simulink model "ES101A_DiagcMgr"  (R2013b)
settings: Solver=ode45  StartTime=0.0  StopTime=0.44  RelTol=1e-3
values from neighbouring files (symbols this model uses):
  BrdgVltg = DataDict.IpSignal    [ES101A_DiagcMgr_DataDict.m]
  DEM_CLEAR_PENDING = DataDict.Constant    [ES101A_DiagcMgr_DataDict.m]
  DEM_DTC_GROUP_ALL_DTCS = DataDict.Constant    [ES101A_DiagcMgr_DataDict.m]
  DFTAGICNTR_CNT_U08 = DataDict.Constant    [ES101A_DiagcMgr_DataDict.m]
  DIAGCMGR_NTCINFOSTSTESTFAILD_CNT_U08 = DataDict.Constant    [ES101A_DiagcMgr_DataDict.m]
  DIAGCMGR_NTCINFOSTSTESTFAILDTHISIGNCYC_CNT_U08 = DataDict.Constant    [ES101A_DiagcMgr_DataDict.m]
  DIAGCMGR_NTCINFOSTSTESTNOTCMPLTHISIGNCYC_CNT_U08 = DataDict.Constant    [ES101A_DiagcMgr_DataDict.m]
  DiagcMgrFltResp = DataDict.Calibration    [ES101A_DiagcMgr_DataDict.m]
  DiagcMgrNtcFltAry = DataDict.NVM    [ES101A_DiagcMgr_DataDict.m]
  DIAGCSTSCTRLDSHTDWNFLTPRSNT_CNT_U16 = DataDict.Constant    [ES101A_DiagcMgr_DataDict.m]
  DIAGCSTSDFTHWAG_CNT_U16 = DataDict.Constant    [ES101A_DiagcMgr_DataDict.m]
  DIAGCSTSDFTHWAGSERLCOMEXPRTVAL_CNT_U16 = DataDict.Constant    [ES101A_DiagcMgr_DataDict.m]
  DIAGCSTSDFTVEHSPD_CNT_U16 = DataDict.Constant    [ES101A_DiagcMgr_DataDict.m]
  DIAGCSTSININVAL_CNT_U16 = DataDict.Constant    [ES101A_DiagcMgr_DataDict.m]
  DIAGCSTSIVTR1INACTV_CNT_U16 = DataDict.Constant    [ES101A_DiagcMgr_DataDict.m]
  DIAGCSTSIVTR2INACTV_CNT_U16 = DataDict.Constant    [ES101A_DiagcMgr_DataDict.m]
  DIAGCSTSLIMDTPRFMNC_CNT_U16 = DataDict.Constant    [ES101A_DiagcMgr_DataDict.m]
  DIAGCSTSRAMPTOZEROFLTPRSNT_CNT_U16 = DataDict.Constant    [ES101A_DiagcMgr_DataDict.m]
  DIAGCSTSWHLIMBREJCTNDI_CNT_U16 = DataDict.Constant    [ES101A_DiagcMgr_DataDict.m]
  DTCIDXSTSFAIL_CNT_U08 = DataDict.Constant    [ES101A_DiagcMgr_DataDict.m]
  DTCIDXSTSNONTC_CNT_U08 = DataDict.Constant    [ES101A_DiagcMgr_DataDict.m]
  DTCIDXSTSNORES_CNT_U08 = DataDict.Constant    [ES101A_DiagcMgr_DataDict.m]
  DTCIDXSTSPASS_CNT_U08 = DataDict.Constant    [ES101A_DiagcMgr_DataDict.m]
  DTCIDXSTSUPDCFMD_CNT_U08 = DataDict.Constant    [ES101A_DiagcMgr_DataDict.m]
  ELECGLBPRM_IVTRCNT_CNT_U08 = DataDict.ConfigParam    [ES101A_DiagcMgr_DataDict.m]
  FLTINJ_DIAGCMGR_DIAGCSTSIVTR1INACTV = DataDict.Constant    [ES101A_DiagcMgr_DataDict.m]
  FLTINJ_DIAGCMGR_DIAGCSTSIVTR2INACTV = DataDict.Constant    [ES101A_DiagcMgr_DataDict.m]
  HwTq = DataDict.IpSignal    [ES101A_DiagcMgr_DataDict.m]
  IgnCntr = DataDict.IpSignal    [ES101A_DiagcMgr_DataDict.m]
  MAXDEBCNTRVAL_CNT_S16 = DataDict.Constant    [ES101A_DiagcMgr_DataDict.m]
  MAXRAMPRATE_ULSPERSEC_F32 = DataDict.Constant    [ES101A_DiagcMgr_DataDict.m]
  MINDEBCNTRVAL_CNT_S16 = DataDict.Constant    [ES101A_DiagcMgr_DataDict.m]
  MINRAMPRATE_ULSPERSEC_F32 = DataDict.Constant    [ES101A_DiagcMgr_DataDict.m]
  SCAMOTTQCMDTOONE_ULS_F32 = DataDict.Constant    [ES101A_DiagcMgr_DataDict.m]
  SCAMOTTQCMDTOZERO_ULS_F32 = DataDict.Constant    [ES101A_DiagcMgr_DataDict.m]
  SysSt = DataDict.IpSignal    [ES101A_DiagcMgr_DataDict.m]
  VehSpd = DataDict.IpSignal    [ES101A_DiagcMgr_DataDict.m]
undefined symbols (not defined in the file or in its folder): ActvMotTqCmdSca, ActvRampRate, AgiCntr, Dem_DTCFormatType, Dem_DTCOriginType, Dem_EventStatusType, DiagcData, DiagcMgrNtcMap, DiagcSts, DtcEnaMask, EcuT, HistNtcFltAry, MicroDiagcData, MotTq, NtcNr, NtcNrWithResd1, NtcStInfo, ProxySetNtcData, Sts, SysSt1, TOTNROFDTC_CNT_U08
libraries: simulink x151, FloatToFixd x5, NxtrNvM x4
(part 11 of 13)

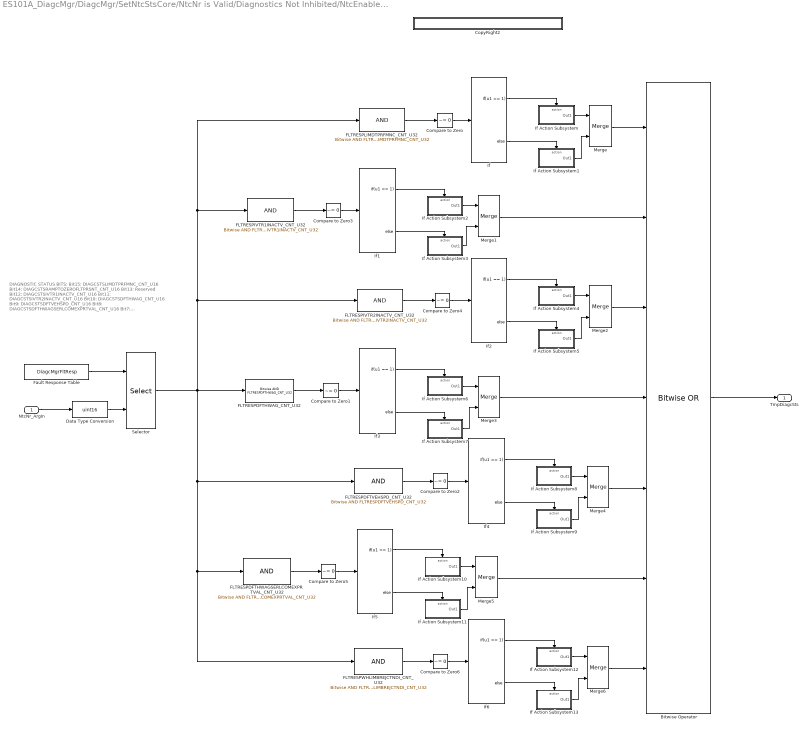
== system ES101A_DiagcMgr/DiagcMgr/SetNtcStsCore/NtcNr is Valid/Diagnostics Not Inhibited/NtcEnabled/NTCSTS_PREFAILD/Update NtcInfoSts, DebCntr and Process RampRate/DebCntr = MAXDEBCNTRVAL_CNT_S16/ProcessRampResponse and DiagcSts/ProcessDiagcSts ==
  note: DIAGNOSTIC  STATUS  BITS:
      |
      | Bit15: DIAGCSTSLIMDTPRFMNC_CNT_U16
      | Bit14: DIAGCSTSRAMPTOZEROFLTPRSNT_CNT_U16
      | Bit13: Reserved
      | Bit12: DIAGCSTSIVTR1INACTV_CNT_U16
      | Bit11: DIAGCSTSIVTR2INACTV_CNT_U16
      | Bit10: DIAGCSTSDFTHWAG_CNT_U16
      | Bit9:   DIAGCSTSDFTVEHSPD_CNT_U16
      | Bit8:   DIAGCSTSDFTHWAGSERLCOMEXPRTVAL_CNT_U16
      | Bit7:   DIAGCSTSWHLIMBREJCTNDI_CNT_U16
      | Bit6:	   DIAGCSTSCTRLDIRAMP_CNT_U16
  NtcNr_ArgIn : Inport
  Bitwise Operator : simulink/Logic and Bit Operations/Bitwise Operator  logicop=OR  UseBitMask=off  NumInputPorts=7  BitMask=bin2dec('11011001')  BitMaskRealWorld=Stored Integer
  Compare to Zero{,1..6} (7 alike) : simulink/Logic and Bit Operations/Compare To Zero  relop=~=  OutDataTypeStr=boolean
  CopyRight2 : Subsystem  Description=|  mask(Copyright Information){none=on}
      | Copyright info block.                                               
      |                                                                     
      | Place copyright information at the top of every subsystem in design.
      mask prompts: none "No parameters"
      mask help: Place copyright information at the top of every subsystem in design.
      mask Display:
      | NxtrConf = 'Nexteer Confidential';
      | 
      | sys = bdroot; %handle for the current model ("system")
      | first = get_param(sys,'Created');
      | first = first(end-3:end);  %year is last four digits
      | 
      | last = get_param(sys,'LastModifiedDate');
      | if isempty(last)
      |     last = datestr(now,'yyyy');
      | else
      |     last = last(end-3:end);
      | end
      | 
      | if strcmp(first,last)
      |     fprintf('%s -- Copyright %s Nexteer',NxtrConf,first)
      | else
      |     fprintf('%s -- %s%s- %s Nexteer',NxtrConf,char(169),first,last)
      | end
  Data Type Conversion : DataTypeConversion  OutDataTypeStr=uint16
  FLTRESPDFTHWAGSERLCOMEXPRTVAL_CNT_U32 : simulink/Logic and Bit Operations/Bitwise Operator  logicop=AND  UseBitMask=on  BitMask=FLTRESPDFTHWAGSERLCOMEXPRTVAL_CNT_U32  BitMaskRealWorld=Stored Integer
  FLTRESPDFTHWAG_CNT_U32 : simulink/Logic and Bit Operations/Bitwise Operator  logicop=AND  UseBitMask=on  BitMask=FLTRESPDFTHWAG_CNT_U32  BitMaskRealWorld=Stored Integer
  FLTRESPDFTVEHSPD_CNT_U32 : simulink/Logic and Bit Operations/Bitwise Operator  logicop=AND  UseBitMask=on  BitMask=FLTRESPDFTVEHSPD_CNT_U32  BitMaskRealWorld=Stored Integer
  FLTRESPIVTR1INACTV_CNT_U32 : simulink/Logic and Bit Operations/Bitwise Operator  RequirementInfo={} %GIDa_0bcc46f0_a928_4871_ba10_4f644a1952a4  logicop=AND  UseBitMask=on  BitMask=FLTRESPIVTR1INACTV_CNT_U32  BitMaskRealWorld=Stored Integer
  FLTRESPIVTR2INACTV_CNT_U32 : simulink/Logic and Bit Operations/Bitwise Operator  RequirementInfo={} %GIDa_28fb51b4_ae96_48d8_a363_96275df46548  logicop=AND  UseBitMask=on  BitMask=FLTRESPIVTR2INACTV_CNT_U32  BitMaskRealWorld=Stored Integer
  FLTRESPLIMDTPRFMNC_CNT_U32 : simulink/Logic and Bit Operations/Bitwise Operator  RequirementInfo={} %GIDa_963dc497_cc80_465d_aac9_827ad747b599  logicop=AND  UseBitMask=on  BitMask=FLTRESPLIMDTPRFMNC_CNT_U32  BitMaskRealWorld=Stored Integer
  FLTRESPWHLIMBREJCTNDI_CNT_U32 : simulink/Logic and Bit Operations/Bitwise Operator  logicop=AND  UseBitMask=on  BitMask=FLTRESPWHLIMBREJCTNDI_CNT_U32  BitMaskRealWorld=Stored Integer
  Fault Response Table : Constant  Value=DiagcMgrFltResp
  If{,1..6} (7 alike) : If  IfExpression=u1 == 1
  If Action Subsystem : Subsystem  TreatAsAtomicUnit=on
  If Action Subsystem1 : Subsystem  TreatAsAtomicUnit=on
  If Action Subsystem10 : Subsystem  TreatAsAtomicUnit=on
  If Action Subsystem11 : Subsystem  TreatAsAtomicUnit=on
  If Action Subsystem12 : Subsystem  TreatAsAtomicUnit=on
  If Action Subsystem13 : Subsystem  TreatAsAtomicUnit=on
  If Action Subsystem2 : Subsystem  TreatAsAtomicUnit=on
  If Action Subsystem3 : Subsystem  TreatAsAtomicUnit=on
  If Action Subsystem4 : Subsystem  TreatAsAtomicUnit=on
  If Action Subsystem5 : Subsystem  TreatAsAtomicUnit=on
  If Action Subsystem6 : Subsystem  TreatAsAtomicUnit=on
  If Action Subsystem7 : Subsystem  TreatAsAtomicUnit=on
  If Action Subsystem8 : Subsystem  TreatAsAtomicUnit=on
  If Action Subsystem9 : Subsystem  TreatAsAtomicUnit=on
  Merge{,1..6} (7 alike) : Merge
  Selector : Selector  IndexMode=Zero-based  InputPortWidth=512  IndexOptions=Index vector (port)  Indices=[1 3]  OutputSizes=1
  TmpDiagcSts : Outport
  wires:
  Compare to Zero4/1 -> If2/1
  Merge2/1 -> Bitwise Operator/3
  If Action Subsystem5/1(Out1) -> Merge2/2
  If Action Subsystem4/1(Out1) -> Merge2/1
  If2/2 -> If Action Subsystem5/Action
  If2/1 -> If Action Subsystem4/Action
  Merge1/1 -> Bitwise Operator/2
  Compare to Zero3/1 -> If1/1
  If Action Subsystem3/1(Out1) -> Merge1/2
  If Action Subsystem2/1(Out1) -> Merge1/1
  If1/2 -> If Action Subsystem3/Action
  If1/1 -> If Action Subsystem2/Action
  Merge/1 -> Bitwise Operator/1
  If Action Subsystem1/1(Out1) -> Merge/2
  If Action Subsystem/1(Out1) -> Merge/1
  Compare to Zero/1 -> If/1
  If/2 -> If Action Subsystem1/Action
  If/1 -> If Action Subsystem/Action
  Bitwise Operator/1 -> TmpDiagcSts/1
  FLTRESPIVTR2INACTV_CNT_U32/1 -> Compare to Zero4/1
  FLTRESPIVTR1INACTV_CNT_U32/1 -> Compare to Zero3/1
  Selector/1 -> FLTRESPWHLIMBREJCTNDI_CNT_U32/1, FLTRESPDFTHWAGSERLCOMEXPRTVAL_CNT_U32/1, FLTRESPDFTVEHSPD_CNT_U32/1, FLTRESPDFTHWAG_CNT_U32/1, FLTRESPLIMDTPRFMNC_CNT_U32/1, FLTRESPIVTR1INACTV_CNT_U32/1, FLTRESPIVTR2INACTV_CNT_U32/1
  Fault Response Table/1 -> Selector/1
  NtcNr_ArgIn/1 -> Data Type Conversion/1
  FLTRESPLIMDTPRFMNC_CNT_U32/1 -> Compare to Zero/1
  Compare to Zero1/1 -> If3/1
  Merge3/1 -> Bitwise Operator/4
  If Action Subsystem7/1(Out1) -> Merge3/2
  If Action Subsystem6/1(Out1) -> Merge3/1
  If3/2 -> If Action Subsystem7/Action
  If3/1 -> If Action Subsystem6/Action
  FLTRESPDFTHWAG_CNT_U32/1 -> Compare to Zero1/1
  Compare to Zero2/1 -> If4/1
  Merge4/1 -> Bitwise Operator/5
  If Action Subsystem9/1(Out1) -> Merge4/2
  If Action Subsystem8/1(Out1) -> Merge4/1
  If4/2 -> If Action Subsystem9/Action
  If4/1 -> If Action Subsystem8/Action
  FLTRESPDFTVEHSPD_CNT_U32/1 -> Compare to Zero2/1
  Compare to Zero5/1 -> If5/1
  Merge5/1 -> Bitwise Operator/6
  If Action Subsystem11/1(Out1) -> Merge5/2
  If Action Subsystem10/1(Out1) -> Merge5/1
  If5/2 -> If Action Subsystem11/Action
  If5/1 -> If Action Subsystem10/Action
  FLTRESPDFTHWAGSERLCOMEXPRTVAL_CNT_U32/1 -> Compare to Zero5/1
  Compare to Zero6/1 -> If6/1
  Merge6/1 -> Bitwise Operator/7
  If Action Subsystem13/1(Out1) -> Merge6/2
  If Action Subsystem12/1(Out1) -> Merge6/1
  If6/2 -> If Action Subsystem13/Action
  If6/1 -> If Action Subsystem12/Action
  FLTRESPWHLIMBREJCTNDI_CNT_U32/1 -> Compare to Zero6/1
  Data Type Conversion/1 -> Selector/2

== system ES101A_DiagcMgr/DiagcMgr/SetNtcStsCore/NtcNr is Valid/Diagnostics Not Inhibited/NtcEnabled/NTCSTS_PREFAILD/Update NtcInfoSts, DebCntr and Process RampRate/DebCntr = MAXDEBCNTRVAL_CNT_S16/ProcessRampResponse and DiagcSts/RapidShutdown Fault ==
  DiagcData_ArgInOut : Inport
  ProxySetNtcData_ArgInOut : Inport  Port=2
  TmpDiagcSts : Inport  Port=3
  Action Port : ActionPort
  Atomic Section2 : Subsystem  Description=|  RequirementInfo="{'linktype_rmi_doors' '0000c474 (/ESG Group/FDD Module Requirements/EA4 Specific/ES101A_DiagcMgr)' '#ES101A_300' 'true' 'REQ:  ES101A_300' '' } %GIDa_f530f53f_5973_437e_b832_6bd1eb8b580f"
      | EXCLUSIVE AREA:
      | Write data into the DiagcSts Register & ActvRampRate Register
      settings: AttributesFormatString=%<Description>
  Bitwise Operator : simulink/Logic and Bit Operations/Bitwise Operator  logicop=OR  UseBitMask=off  NumInputPorts=2  BitMask=bin2dec('11011001')  BitMaskRealWorld=Stored Integer
  CopyRight2 : Subsystem  Description=|  mask(Copyright Information){none=on}
      | Copyright info block.                                               
      |                                                                     
      | Place copyright information at the top of every subsystem in design.
      mask prompts: none "No parameters"
      mask help: Place copyright information at the top of every subsystem in design.
      mask Display:
      | NxtrConf = 'Nexteer Confidential';
      | 
      | sys = bdroot; %handle for the current model ("system")
      | first = get_param(sys,'Created');
      | first = first(end-3:end);  %year is last four digits
      | 
      | last = get_param(sys,'LastModifiedDate');
      | if isempty(last)
      |     last = datestr(now,'yyyy');
      | else
      |     last = last(end-3:end);
      | end
      | 
      | if strcmp(first,last)
      |     fprintf('%s -- Copyright %s Nexteer',NxtrConf,first)
      | else
      |     fprintf('%s -- %s%s- %s Nexteer',NxtrConf,char(169),first,last)
      | end
  Ramp To Zero Fault Present1 : Constant  Value=DIAGCSTSRAMPTOZEROFLTPRSNT_CNT_U16  OutDataTypeStr=uint16
  DiagcData_ArgOut : Outport
  ProxySetNtcData_ArgOut : Outport  Port=2
  wires:
  Ramp To Zero Fault Present1/1 -> Bitwise Operator/1
  Bitwise Operator/1 -> Atomic Section2/1(TmpDiagcSts)
  TmpDiagcSts/1 -> Bitwise Operator/2
  DiagcData_ArgInOut/1 -> Atomic Section2/2(DiagcData_ArgInOut)
  ProxySetNtcData_ArgInOut/1 -> Atomic Section2/3(ProxySetNtcData_ArgInOut)
  Atomic Section2/1(DiagcData_ArgOut) -> DiagcData_ArgOut/1
  Atomic Section2/2(ProxySetNtcData_ArgOut) -> ProxySetNtcData_ArgOut/1

== system ES101A_DiagcMgr/DiagcMgr/SetNtcStsCore/NtcNr is Valid/Diagnostics Not Inhibited/NtcEnabled/NTCSTS_PREFAILD/Update NtcInfoSts, DebCntr and Process RampRate/DebCntr = MAXDEBCNTRVAL_CNT_S16/ProcessRampResponse and DiagcSts/TimedShutdown Fault ==
  FaultResponseRampBits : Inport
  DiagcData_ArgInOut : Inport  Port=2
  ProxySetNtcData_ArgInOut : Inport  Port=3
  TmpDiagcSts : Inport  Port=4
  Action Port : ActionPort
  Atomic Section2 : Subsystem  Description=|  RequirementInfo="{'linktype_rmi_doors' '0000c474 (/ESG Group/FDD Module Requirements/EA4 Specific/ES101A_DiagcMgr)' '#ES101A_300' 'true' 'REQ:  ES101A_300' '' } %GIDa_6b3329a8_a629_4212_a9db_bb0aaf80cc69"
      | EXCLUSIVE AREA:
      | Write data into the DiagcSts Register & ActvRampRate Register
      settings: AttributesFormatString=%<Description>
  Bitwise Operator : simulink/Logic and Bit Operations/Bitwise Operator  logicop=OR  UseBitMask=off  NumInputPorts=2  BitMask=bin2dec('11011001')  BitMaskRealWorld=Stored Integer
  CopyRight2 : Subsystem  Description=|  mask(Copyright Information){none=on}
      | Copyright info block.                                               
      |                                                                     
      | Place copyright information at the top of every subsystem in design.
      mask prompts: none "No parameters"
      mask help: Place copyright information at the top of every subsystem in design.
      mask Display:
      | NxtrConf = 'Nexteer Confidential';
      | 
      | sys = bdroot; %handle for the current model ("system")
      | first = get_param(sys,'Created');
      | first = first(end-3:end);  %year is last four digits
      | 
      | last = get_param(sys,'LastModifiedDate');
      | if isempty(last)
      |     last = datestr(now,'yyyy');
      | else
      |     last = last(end-3:end);
      | end
      | 
      | if strcmp(first,last)
      |     fprintf('%s -- Copyright %s Nexteer',NxtrConf,first)
      | else
      |     fprintf('%s -- %s%s- %s Nexteer',NxtrConf,char(169),first,last)
      | end
  Direct Lookup Table (n-D)1 : LookupNDDirect  NumberOfTableDimensions=1  Table=[0.1,0.125,0.1428,0.1667,0.2,0.25,0.333,0.5,1,2,3.333,10,500]  TableDataTypeStr=single
  Ramp To Zero Fault Present : Constant  Value=DIAGCSTSRAMPTOZEROFLTPRSNT_CNT_U16  OutDataTypeStr=uint16
  DiagcData_ArgOut : Outport
  ProxySetNtcData_ArgOut : Outport  Port=2
  wires:
  Ramp To Zero Fault Present/1 -> Bitwise Operator/1
  TmpDiagcSts/1 -> Bitwise Operator/2
  FaultResponseRampBits/1 -> Direct Lookup Table (n-D)1/1
  Direct Lookup Table (n-D)1/1 -> Atomic Section2/2(RampRate)
  Atomic Section2/1(DiagcData_ArgOut) -> DiagcData_ArgOut/1
  Atomic Section2/2(ProxySetNtcData_ArgOut) -> ProxySetNtcData_ArgOut/1
  Bitwise Operator/1 -> Atomic Section2/1(TmpDiagcSts)
  DiagcData_ArgInOut/1 -> Atomic Section2/3(DiagcData_ArgInOut)
  ProxySetNtcData_ArgInOut/1 -> Atomic Section2/4(ProxySetNtcData_ArgInOut)

== system ES101A_DiagcMgr/DiagcMgr/SetNtcStsCore/NtcNr is Valid/Diagnostics Not Inhibited/NtcEnabled/NTCSTS_PREFAILD/Update NtcInfoSts, DebCntr and Process RampRate/DebCntr = MAXDEBCNTRVAL_CNT_S16/Update NtcSts and DebCntr/Clear: DIAGCMGR_NTCINFOSTSTESTNOTCMPLTHISIGNCYC_CNT_U08 ==
  In2 : Inport
  In1 : Inport  Port=2
  Bitwise Operator : simulink/Logic and Bit Operations/Bitwise Operator  logicop=NOT  UseBitMask=off  BitMask=bin2dec('11011001')  BitMaskRealWorld=Stored Integer
  Bitwise Operator1 : simulink/Logic and Bit Operations/Bitwise Operator  logicop=AND  UseBitMask=off  NumInputPorts=2  BitMask=bin2dec('11011001')  BitMaskRealWorld=Stored Integer
  Out1 : Outport
  wires:
  Bitwise Operator1/1 -> Out1/1
  In2/1 -> Bitwise Operator1/1
  In1/1 -> Bitwise Operator/1
  Bitwise Operator/1 -> Bitwise Operator1/2

== system ES101A_DiagcMgr/DiagcMgr/SetNtcStsCore/NtcNr is Valid/Diagnostics Not Inhibited/NtcEnabled/NTCSTS_PREFAILD/Update NtcInfoSts, DebCntr and Process RampRate/DebCntr = MAXDEBCNTRVAL_CNT_S16/Update NtcSts and DebCntr/Copyright1 ==

== system ES101A_DiagcMgr/DiagcMgr/SetNtcStsCore/NtcNr is Valid/Diagnostics Not Inhibited/NtcEnabled/NTCSTS_PREPASSD/Update NtcInfoSts/Update NTC Info's Status Byte & Update the NTC Fault Array/Decrement Counter/Copyright1 ==

== system ES101A_DiagcMgr/DiagcMgr/SetNtcStsCore/NtcNr is Valid/Diagnostics Not Inhibited/NtcEnabled/NTCSTS_PREPASSD/Update NtcInfoSts/Update NTC Info's Status Byte & Update the NTC Fault Array/Decrement Counter/Deb Counter > MINDEBCNTRVAL_CNT_S16 ==
  DebStep : Inport
  NtcInfoDebCntr_ArgIn : Inport  Port=2
  Action Port : ActionPort
  Copyright1 : Subsystem  Description=|  mask(Copyright Information){none=on}
      | Copyright info block.                                               
      |                                                                     
      | Place copyright information at the top of every subsystem in design.
      mask prompts: none "No parameters"
      mask help: Place copyright information at the top of every subsystem in design.
      mask Display:
      | NxtrConf = 'Nexteer Confidential';
      | 
      | sys = bdroot; %handle for the current model ("system")
      | first = get_param(sys,'Created');
      | if(isempty(first))
      |     first = datestr(now,'yyyy');
      | else
      |     first = first(end-3:end);  %year is last four digits
      | end
      | 
      | last = get_param(sys,'LastModifiedDate');
      | if isempty(last)
      |     last = datestr(now,'yyyy');
      | else
      |     last = last(end-3:end);
      | end
      | 
      | if strcmp(first,last)
      |     fprintf('%s\nCopyright  %s Nexteer',NxtrConf,first);
      | else
      |     fprintf('%s\n%s%s-%s Nexteer',NxtrConf,char(169),first,last);
      | end
  Sub : Sum  Inputs=+-  SaturateOnIntegerOverflow=on
  NtcInfoDebCntr_ArgOut : Outport
  wires:
  Sub/1 -> NtcInfoDebCntr_ArgOut/1
  DebStep/1 -> Sub/2
  NtcInfoDebCntr_ArgIn/1 -> Sub/1

== system ES101A_DiagcMgr/DiagcMgr/SetNtcStsCore/NtcNr is Valid/Diagnostics Not Inhibited/NtcEnabled/NTCSTS_PREPASSD/Update NtcInfoSts/Update NTC Info's Status Byte & Update the NTC Fault Array/Decrement Counter/DebCntr = MINDEBCNTRVAL_CNT_S16 ==
  note: Sts not DebCntr
  NtcInfo_ArgIn : Inport
  Action Port : ActionPort
  Bus Assignment1 : BusAssignment  AssignedSignals=Sts
  Bus Selector2 : BusSelector  OutputSignals=DebCntr
  Clear: DIAGCMGR_NTCINFOSTSTESTFAILD_CNT_U08 : Subsystem
  Clear: DIAGCMGR_NTCINFOSTSTESTNOTCMPLTHISIGNCYC_CNT_U08 : Subsystem
  Constant1 : Constant  Value=DIAGCMGR_NTCINFOSTSTESTFAILD_CNT_U08
  Constant2 : Constant  Value=MINDEBCNTRVAL_CNT_S16
  Constant3 : Constant  Value=DIAGCMGR_NTCINFOSTSTESTNOTCMPLTHISIGNCYC_CNT_U08
  Copyright1 : Subsystem  Description=|  mask(Copyright Information){none=on}
      | Copyright info block.                                               
      |                                                                     
      | Place copyright information at the top of every subsystem in design.
      mask prompts: none "No parameters"
      mask help: Place copyright information at the top of every subsystem in design.
      mask Display:
      | NxtrConf = 'Nexteer Confidential';
      | 
      | sys = bdroot; %handle for the current model ("system")
      | first = get_param(sys,'Created');
      | if(isempty(first))
      |     first = datestr(now,'yyyy');
      | else
      |     first = first(end-3:end);  %year is last four digits
      | end
      | 
      | last = get_param(sys,'LastModifiedDate');
      | if isempty(last)
      |     last = datestr(now,'yyyy');
      | else
      |     last = last(end-3:end);
      | end
      | 
      | if strcmp(first,last)
      |     fprintf('%s\nCopyright  %s Nexteer',NxtrConf,first);
      | else
      |     fprintf('%s\n%s%s-%s Nexteer',NxtrConf,char(169),first,last);
      | end
  NtcInfo_ArgOut : Outport
  NtcInfoDebCntr_ArgOut : Outport  Port=2
  wires:
  NtcInfo_ArgIn/1 -> Bus Assignment1/1, Bus Selector2/1
  Constant3/1 -> Clear: DIAGCMGR_NTCINFOSTSTESTNOTCMPLTHISIGNCYC_CNT_U08/2(In1)
  Constant1/1 -> Clear: DIAGCMGR_NTCINFOSTSTESTFAILD_CNT_U08/2(In1)
  Clear: DIAGCMGR_NTCINFOSTSTESTFAILD_CNT_U08/1(Out1) -> Clear: DIAGCMGR_NTCINFOSTSTESTNOTCMPLTHISIGNCYC_CNT_U08/1(In2)
  Bus Selector2/1 -> Clear: DIAGCMGR_NTCINFOSTSTESTFAILD_CNT_U08/1(In2)  "<DebCntr>"
  Bus Assignment1/1 -> NtcInfo_ArgOut/1
  Clear: DIAGCMGR_NTCINFOSTSTESTNOTCMPLTHISIGNCYC_CNT_U08/1(Out1) -> Bus Assignment1/2
  Constant2/1 -> NtcInfoDebCntr_ArgOut/1

== system ES101A_DiagcMgr/DiagcMgr/DiagcMgrPer2/Normal Periodic Processing/For All DTCs/For Each DTC/Check If DTC Status has Changed/DTC Status Changed OR DTC Update NOT Confirmed/Update DTC Status/Dtc Status is Failed/Dem_SetEventStatus/CopyRight2 ==

== system ES101A_DiagcMgr/DiagcMgr/DiagcMgrPer2/Normal Periodic Processing/For All DTCs/For Each DTC/Check If DTC Status has Changed/DTC Status Changed OR DTC Update NOT Confirmed/Update DTC Status/Dtc Status is Failed/Update 'DTC Index Update Confirmed' Bit/CopyRight2 ==

== system ES101A_DiagcMgr/DiagcMgr/DiagcMgrPer2/Normal Periodic Processing/For All DTCs/For Each DTC/Check If DTC Status has Changed/DTC Status Changed OR DTC Update NOT Confirmed/Update DTC Status/Dtc Status is Failed/Update 'DTC Index Update Confirmed' Bit/StdRtn is E_OK ==
  DtcIdx : Inport
  DtcIdxPrevSts : Inport  Port=2
  Action Port : ActionPort
  Assignment : Assignment  IndexMode=Zero-based  IndexOptions=Starting index (port)  Indices=1  OutputSizes=1
  CopyRight2 : Subsystem  Description=|  mask(Copyright Information){none=on}
      | Copyright info block.                                               
      |                                                                     
      | Place copyright information at the top of every subsystem in design.
      mask prompts: none "No parameters"
      mask help: Place copyright information at the top of every subsystem in design.
      mask Display:
      | NxtrConf = 'Nexteer Confidential';
      | 
      | sys = bdroot; %handle for the current model ("system")
      | first = get_param(sys,'Created');
      | first = first(end-3:end);  %year is last four digits
      | 
      | last = get_param(sys,'LastModifiedDate');
      | if isempty(last)
      |     last = datestr(now,'yyyy');
      | else
      |     last = last(end-3:end);
      | end
      | 
      | if strcmp(first,last)
      |     fprintf('%s -- Copyright %s Nexteer',NxtrConf,first)
      | else
      |     fprintf('%s -- %s%s- %s Nexteer',NxtrConf,char(169),first,last)
      | end
  Data Store Read : DataStoreRead  DataStoreName=DtcIdxPrevSts
  Data Store Write : DataStoreWrite  DataStoreName=DtcIdxPrevSts
  Set Bit 7 (DTC Update Confirmed) : Subsystem
  wires:
  Set Bit 7 (DTC Update Confirmed)/1(DtcIdxPrevSts) -> Assignment/2
  DtcIdxPrevSts/1 -> Set Bit 7 (DTC Update Confirmed)/1("DtcIdxPrevSts ")
  DtcIdx/1 -> Assignment/3
  Assignment/1 -> Data Store Write/1
  Data Store Read/1 -> Assignment/1

== system ES101A_DiagcMgr/DiagcMgr/DiagcMgrPer2/Normal Periodic Processing/For All DTCs/For Each DTC/Check If DTC Status has Changed/DTC Status Changed OR DTC Update NOT Confirmed/Update DTC Status/Dtc Status is No Result or No Ntc/Set Bit 7 (DTC Update Confirmed)/CopyRight2 ==

== system ES101A_DiagcMgr/DiagcMgr/DiagcMgrPer2/Normal Periodic Processing/For All DTCs/For Each DTC/Check If DTC Status has Changed/DTC Status Changed OR DTC Update NOT Confirmed/Update DTC Status/Dtc Status is Passed/Dem_SetEventStatus/CopyRight2 ==

== system ES101A_DiagcMgr/DiagcMgr/DiagcMgrPer2/Normal Periodic Processing/For All DTCs/For Each DTC/Check If DTC Status has Changed/DTC Status Changed OR DTC Update NOT Confirmed/Update DTC Status/Dtc Status is Passed/Update 'DTC Index Update Confirmed' Bit/CopyRight2 ==

== system ES101A_DiagcMgr/DiagcMgr/DiagcMgrPer2/Normal Periodic Processing/For All DTCs/For Each DTC/Check If DTC Status has Changed/DTC Status Changed OR DTC Update NOT Confirmed/Update DTC Status/Dtc Status is Passed/Update 'DTC Index Update Confirmed' Bit/StdRtn is E_OK ==
  DtcIdx : Inport
  DtcIdxPrevSts : Inport  Port=2
  Action Port : ActionPort
  Assignment : Assignment  IndexMode=Zero-based  IndexOptions=Starting index (port)  Indices=1  OutputSizes=1
  CopyRight2 : Subsystem  Description=|  mask(Copyright Information){none=on}
      | Copyright info block.                                               
      |                                                                     
      | Place copyright information at the top of every subsystem in design.
      mask prompts: none "No parameters"
      mask help: Place copyright information at the top of every subsystem in design.
      mask Display:
      | NxtrConf = 'Nexteer Confidential';
      | 
      | sys = bdroot; %handle for the current model ("system")
      | first = get_param(sys,'Created');
      | first = first(end-3:end);  %year is last four digits
      | 
      | last = get_param(sys,'LastModifiedDate');
      | if isempty(last)
      |     last = datestr(now,'yyyy');
      | else
      |     last = last(end-3:end);
      | end
      | 
      | if strcmp(first,last)
      |     fprintf('%s -- Copyright %s Nexteer',NxtrConf,first)
      | else
      |     fprintf('%s -- %s%s- %s Nexteer',NxtrConf,char(169),first,last)
      | end
  Data Store Read : DataStoreRead  DataStoreName=DtcIdxPrevSts
  Data Store Write : DataStoreWrite  DataStoreName=DtcIdxPrevSts
  Set Bit 7 (DTC Update Confirmed) : Subsystem
  wires:
  Data Store Read/1 -> Assignment/1
  Assignment/1 -> Data Store Write/1
  DtcIdx/1 -> Assignment/3
  DtcIdxPrevSts/1 -> Set Bit 7 (DTC Update Confirmed)/1("DtcIdxPrevSts ")
  Set Bit 7 (DTC Update Confirmed)/1(DtcIdxPrevSts) -> Assignment/2

== system ES101A_DiagcMgr/DiagcMgr/SetNtcStsCore/NtcNr is Valid/Diagnostics Not Inhibited/NtcEnabled/NTCSTS_FAILD/Update ISO Bits, Parameter Byte and AgiCntr /Check to Update Snapshot Data/UpdSnpshtData/Snapshot Data Enabled/CopyRight2 ==

== system ES101A_DiagcMgr/DiagcMgr/SetNtcStsCore/NtcNr is Valid/Diagnostics Not Inhibited/NtcEnabled/NTCSTS_FAILD/Update ISO Bits, Parameter Byte and AgiCntr /Check to Update Snapshot Data/UpdSnpshtData/Snapshot Data Enabled/Initialize ==
  Constant : Constant  OutDataTypeStr=boolean
  Constant1 : Constant  Value=0  OutDataTypeStr=uint8
  CopyRight2 : Subsystem  Description=|  mask(Copyright Information){none=on}
      | Copyright info block.                                               
      |                                                                     
      | Place copyright information at the top of every subsystem in design.
      mask prompts: none "No parameters"
      mask help: Place copyright information at the top of every subsystem in design.
      mask Display:
      | NxtrConf = 'Nexteer Confidential';
      | 
      | sys = bdroot; %handle for the current model ("system")
      | first = get_param(sys,'Created');
      | first = first(end-3:end);  %year is last four digits
      | 
      | last = get_param(sys,'LastModifiedDate');
      | if isempty(last)
      |     last = datestr(now,'yyyy');
      | else
      |     last = last(end-3:end);
      | end
      | 
      | if strcmp(first,last)
      |     fprintf('%s -- Copyright %s Nexteer',NxtrConf,first)
      | else
      |     fprintf('%s -- %s%s- %s Nexteer',NxtrConf,char(169),first,last)
      | end
  Data Store Write : DataStoreWrite  DataStoreName=SnpshtDataAryIdxInvld
  Data Store Write1 : DataStoreWrite  DataStoreName=SnpshtDataAryIdx
  wires:
  Constant1/1 -> Data Store Write1/1
  Constant/1 -> Data Store Write/1

== system ES101A_DiagcMgr/DiagcMgr/SetNtcStsCore/NtcNr is Valid/Diagnostics Not Inhibited/NtcEnabled/NTCSTS_FAILD/Update ISO Bits, Parameter Byte and AgiCntr /Check to Update Snapshot Data/UpdSnpshtData/Snapshot Data Enabled/While  ==
  NtcNr : Inport
  NtcStInfo : Inport  Port=2
  SnapshotDataBus : Inport  Port=3
  CopyRight2 : Subsystem  Description=|  mask(Copyright Information){none=on}
      | Copyright info block.                                               
      |                                                                     
      | Place copyright information at the top of every subsystem in design.
      mask prompts: none "No parameters"
      mask help: Place copyright information at the top of every subsystem in design.
      mask Display:
      | NxtrConf = 'Nexteer Confidential';
      | 
      | sys = bdroot; %handle for the current model ("system")
      | first = get_param(sys,'Created');
      | first = first(end-3:end);  %year is last four digits
      | 
      | last = get_param(sys,'LastModifiedDate');
      | if isempty(last)
      |     last = datestr(now,'yyyy');
      | else
      |     last = last(end-3:end);
      | end
      | 
      | if strcmp(first,last)
      |     fprintf('%s -- Copyright %s Nexteer',NxtrConf,first)
      | else
      |     fprintf('%s -- %s%s- %s Nexteer',NxtrConf,char(169),first,last)
      | end
  Logical Operator : Logic  AllPortsSameDT=off  OutDataTypeStr=boolean
  Relational Operator : RelationalOperator  Operator=<  OutDataTypeStr=boolean
  Snapshot Data Array : DataStoreRead  DataStoreName=SnpShtDataAry
  Snapshot Data Array Index : DataStoreRead  DataStoreName=SnpshtDataAryIdx
  Snapshot Data Array Index Invalid : DataStoreRead  DataStoreName=SnpshtDataAryIdxInvld
  While NTC Matches or Run out of Index : Subsystem  Priority=2  TreatAsAtomicUnit=on
      settings: AttributesFormatString=Priority = %<Priority>
  Width : Width
  wires:
  Width/1 -> Relational Operator/2
  Logical Operator/1 -> While NTC Matches or Run out of Index/1(IC), While NTC Matches or Run out of Index/2(cond)
  Snapshot Data Array Index Invalid/1 -> Logical Operator/1
  Relational Operator/1 -> Logical Operator/2
  Snapshot Data Array Index/1 -> Relational Operator/1
  Snapshot Data Array/1 -> Width/1
  SnapshotDataBus/1 -> While NTC Matches or Run out of Index/5(SnapshotDataBus)
  NtcStInfo/1 -> While NTC Matches or Run out of Index/4(NtcStInfo)
  NtcNr/1 -> While NTC Matches or Run out of Index/3(NtcNr)

== system ES101A_DiagcMgr/DiagcMgr/SetNtcStsCore/NtcNr is Valid/Diagnostics Not Inhibited/NtcEnabled/NTCSTS_FAILD/Update ISO Bits, Parameter Byte and AgiCntr /ProcessRampResponse and DiagcSts/ControlledShutdown Fault/Atomic Section2/CopyRight2 ==

== system ES101A_DiagcMgr/DiagcMgr/SetNtcStsCore/NtcNr is Valid/Diagnostics Not Inhibited/NtcEnabled/NTCSTS_FAILD/Update ISO Bits, Parameter Byte and AgiCntr /ProcessRampResponse and DiagcSts/ControlledShutdown Fault/Atomic Section2/Update Scale ==
  Action Port : ActionPort
  CopyRight2 : Subsystem  Description=|  mask(Copyright Information){none=on}
      | Copyright info block.                                               
      |                                                                     
      | Place copyright information at the top of every subsystem in design.
      mask prompts: none "No parameters"
      mask help: Place copyright information at the top of every subsystem in design.
      mask Display:
      | NxtrConf = 'Nexteer Confidential';
      | 
      | sys = bdroot; %handle for the current model ("system")
      | first = get_param(sys,'Created');
      | first = first(end-3:end);  %year is last four digits
      | 
      | last = get_param(sys,'LastModifiedDate');
      | if isempty(last)
      |     last = datestr(now,'yyyy');
      | else
      |     last = last(end-3:end);
      | end
      | 
      | if strcmp(first,last)
      |     fprintf('%s -- Copyright %s Nexteer',NxtrConf,first)
      | else
      |     fprintf('%s -- %s%s- %s Nexteer',NxtrConf,char(169),first,last)
      | end
  Scale Motor Torque Command to Zero : Constant  Value=SCAMOTTQCMDTOZERO_ULS_F32  OutDataTypeStr=single
  DiagcMgrActvMotTqCmdSca : Outport
  wires:
  Scale Motor Torque Command to Zero/1 -> DiagcMgrActvMotTqCmdSca/1

== system ES101A_DiagcMgr/DiagcMgr/SetNtcStsCore/NtcNr is Valid/Diagnostics Not Inhibited/NtcEnabled/NTCSTS_FAILD/Update ISO Bits, Parameter Byte and AgiCntr /ProcessRampResponse and DiagcSts/ControlledShutdown Fault/Atomic Section2/Update Scale1 ==
  Action Port : ActionPort
  CopyRight2 : Subsystem  Description=|  mask(Copyright Information){none=on}
      | Copyright info block.                                               
      |                                                                     
      | Place copyright information at the top of every subsystem in design.
      mask prompts: none "No parameters"
      mask help: Place copyright information at the top of every subsystem in design.
      mask Display:
      | NxtrConf = 'Nexteer Confidential';
      | 
      | sys = bdroot; %handle for the current model ("system")
      | first = get_param(sys,'Created');
      | first = first(end-3:end);  %year is last four digits
      | 
      | last = get_param(sys,'LastModifiedDate');
      | if isempty(last)
      |     last = datestr(now,'yyyy');
      | else
      |     last = last(end-3:end);
      | end
      | 
      | if strcmp(first,last)
      |     fprintf('%s -- Copyright %s Nexteer',NxtrConf,first)
      | else
      |     fprintf('%s -- %s%s- %s Nexteer',NxtrConf,char(169),first,last)
      | end
  Scale Motor Torque Command to Zero : Constant  Value=SCAMOTTQCMDTOZERO_ULS_F32  OutDataTypeStr=single
  ProxySetNtcMotTqCmdSca : Outport
  wires:
  Scale Motor Torque Command to Zero/1 -> ProxySetNtcMotTqCmdSca/1

== system ES101A_DiagcMgr/DiagcMgr/SetNtcStsCore/NtcNr is Valid/Diagnostics Not Inhibited/NtcEnabled/NTCSTS_FAILD/Update ISO Bits, Parameter Byte and AgiCntr /ProcessRampResponse and DiagcSts/InformationOnly Fault/Atomic Section2/CopyRight2 ==

== system ES101A_DiagcMgr/DiagcMgr/SetNtcStsCore/NtcNr is Valid/Diagnostics Not Inhibited/NtcEnabled/NTCSTS_FAILD/Update ISO Bits, Parameter Byte and AgiCntr /ProcessRampResponse and DiagcSts/RapidShutdown Fault/Atomic Section2/CopyRight2 ==

== system ES101A_DiagcMgr/DiagcMgr/SetNtcStsCore/NtcNr is Valid/Diagnostics Not Inhibited/NtcEnabled/NTCSTS_FAILD/Update ISO Bits, Parameter Byte and AgiCntr /ProcessRampResponse and DiagcSts/RapidShutdown Fault/Atomic Section2/Update Ramp Rate ==
  Action Port : ActionPort
  CopyRight2 : Subsystem  Description=|  mask(Copyright Information){none=on}
      | Copyright info block.                                               
      |                                                                     
      | Place copyright information at the top of every subsystem in design.
      mask prompts: none "No parameters"
      mask help: Place copyright information at the top of every subsystem in design.
      mask Display:
      | NxtrConf = 'Nexteer Confidential';
      | 
      | sys = bdroot; %handle for the current model ("system")
      | first = get_param(sys,'Created');
      | first = first(end-3:end);  %year is last four digits
      | 
      | last = get_param(sys,'LastModifiedDate');
      | if isempty(last)
      |     last = datestr(now,'yyyy');
      | else
      |     last = last(end-3:end);
      | end
      | 
      | if strcmp(first,last)
      |     fprintf('%s -- Copyright %s Nexteer',NxtrConf,first)
      | else
      |     fprintf('%s -- %s%s- %s Nexteer',NxtrConf,char(169),first,last)
      | end
  Maximum Ramp Rate : Constant  Value=MAXRAMPRATE_ULSPERSEC_F32  OutDataTypeStr=single
  DiagcMgrActvRampRate : Outport
  wires:
  Maximum Ramp Rate/1 -> DiagcMgrActvRampRate/1

== system ES101A_DiagcMgr/DiagcMgr/SetNtcStsCore/NtcNr is Valid/Diagnostics Not Inhibited/NtcEnabled/NTCSTS_FAILD/Update ISO Bits, Parameter Byte and AgiCntr /ProcessRampResponse and DiagcSts/RapidShutdown Fault/Atomic Section2/Update Ramp Rate1 ==
  Action Port : ActionPort
  CopyRight2 : Subsystem  Description=|  mask(Copyright Information){none=on}
      | Copyright info block.                                               
      |                                                                     
      | Place copyright information at the top of every subsystem in design.
      mask prompts: none "No parameters"
      mask help: Place copyright information at the top of every subsystem in design.
      mask Display:
      | NxtrConf = 'Nexteer Confidential';
      | 
      | sys = bdroot; %handle for the current model ("system")
      | first = get_param(sys,'Created');
      | first = first(end-3:end);  %year is last four digits
      | 
      | last = get_param(sys,'LastModifiedDate');
      | if isempty(last)
      |     last = datestr(now,'yyyy');
      | else
      |     last = last(end-3:end);
      | end
      | 
      | if strcmp(first,last)
      |     fprintf('%s -- Copyright %s Nexteer',NxtrConf,first)
      | else
      |     fprintf('%s -- %s%s- %s Nexteer',NxtrConf,char(169),first,last)
      | end
  Maximum Ramp Rate : Constant  Value=MAXRAMPRATE_ULSPERSEC_F32  OutDataTypeStr=single
  ProxySetNtcActvRampRate : Outport
  wires:
  Maximum Ramp Rate/1 -> ProxySetNtcActvRampRate/1

== system ES101A_DiagcMgr/DiagcMgr/SetNtcStsCore/NtcNr is Valid/Diagnostics Not Inhibited/NtcEnabled/NTCSTS_FAILD/Update ISO Bits, Parameter Byte and AgiCntr /ProcessRampResponse and DiagcSts/RapidShutdown Fault/Atomic Section2/Update Scale2 ==
  Action Port : ActionPort
  CopyRight2 : Subsystem  Description=|  mask(Copyright Information){none=on}
      | Copyright info block.                                               
      |                                                                     
      | Place copyright information at the top of every subsystem in design.
      mask prompts: none "No parameters"
      mask help: Place copyright information at the top of every subsystem in design.
      mask Display:
      | NxtrConf = 'Nexteer Confidential';
      | 
      | sys = bdroot; %handle for the current model ("system")
      | first = get_param(sys,'Created');
      | first = first(end-3:end);  %year is last four digits
      | 
      | last = get_param(sys,'LastModifiedDate');
      | if isempty(last)
      |     last = datestr(now,'yyyy');
      | else
      |     last = last(end-3:end);
      | end
      | 
      | if strcmp(first,last)
      |     fprintf('%s -- Copyright %s Nexteer',NxtrConf,first)
      | else
      |     fprintf('%s -- %s%s- %s Nexteer',NxtrConf,char(169),first,last)
      | end
  Scale Motor Torque Command to Zero : Constant  Value=SCAMOTTQCMDTOZERO_ULS_F32  OutDataTypeStr=single
  DiagcMgrActvMotTqCmdSca : Outport
  wires:
  Scale Motor Torque Command to Zero/1 -> DiagcMgrActvMotTqCmdSca/1

== system ES101A_DiagcMgr/DiagcMgr/SetNtcStsCore/NtcNr is Valid/Diagnostics Not Inhibited/NtcEnabled/NTCSTS_FAILD/Update ISO Bits, Parameter Byte and AgiCntr /ProcessRampResponse and DiagcSts/RapidShutdown Fault/Atomic Section2/Update Scale3 ==
  Action Port : ActionPort
  CopyRight2 : Subsystem  Description=|  mask(Copyright Information){none=on}
      | Copyright info block.                                               
      |                                                                     
      | Place copyright information at the top of every subsystem in design.
      mask prompts: none "No parameters"
      mask help: Place copyright information at the top of every subsystem in design.
      mask Display:
      | NxtrConf = 'Nexteer Confidential';
      | 
      | sys = bdroot; %handle for the current model ("system")
      | first = get_param(sys,'Created');
      | first = first(end-3:end);  %year is last four digits
      | 
      | last = get_param(sys,'LastModifiedDate');
      | if isempty(last)
      |     last = datestr(now,'yyyy');
      | else
      |     last = last(end-3:end);
      | end
      | 
      | if strcmp(first,last)
      |     fprintf('%s -- Copyright %s Nexteer',NxtrConf,first)
      | else
      |     fprintf('%s -- %s%s- %s Nexteer',NxtrConf,char(169),first,last)
      | end
  Scale Motor Torque Command to Zero : Constant  Value=SCAMOTTQCMDTOZERO_ULS_F32  OutDataTypeStr=single
  ProxySetNtcMotTqCmdSca : Outport
  wires:
  Scale Motor Torque Command to Zero/1 -> ProxySetNtcMotTqCmdSca/1

== system ES101A_DiagcMgr/DiagcMgr/SetNtcStsCore/NtcNr is Valid/Diagnostics Not Inhibited/NtcEnabled/NTCSTS_FAILD/Update ISO Bits, Parameter Byte and AgiCntr /ProcessRampResponse and DiagcSts/TimedShutdown Fault/Atomic Section2/CopyRight2 ==

== system ES101A_DiagcMgr/DiagcMgr/SetNtcStsCore/NtcNr is Valid/Diagnostics Not Inhibited/NtcEnabled/NTCSTS_FAILD/Update ISO Bits, Parameter Byte and AgiCntr /ProcessRampResponse and DiagcSts/TimedShutdown Fault/Atomic Section2/Update Ramp Rate ==
  RampRate : Inport
  Action Port : ActionPort
  CopyRight2 : Subsystem  Description=|  mask(Copyright Information){none=on}
      | Copyright info block.                                               
      |                                                                     
      | Place copyright information at the top of every subsystem in design.
      mask prompts: none "No parameters"
      mask help: Place copyright information at the top of every subsystem in design.
      mask Display:
      | NxtrConf = 'Nexteer Confidential';
      | 
      | sys = bdroot; %handle for the current model ("system")
      | first = get_param(sys,'Created');
      | first = first(end-3:end);  %year is last four digits
      | 
      | last = get_param(sys,'LastModifiedDate');
      | if isempty(last)
      |     last = datestr(now,'yyyy');
      | else
      |     last = last(end-3:end);
      | end
      | 
      | if strcmp(first,last)
      |     fprintf('%s -- Copyright %s Nexteer',NxtrConf,first)
      | else
      |     fprintf('%s -- %s%s- %s Nexteer',NxtrConf,char(169),first,last)
      | end
  DiagcMgrActvRampRate : Outport
  wires:
  RampRate/1 -> DiagcMgrActvRampRate/1

== system ES101A_DiagcMgr/DiagcMgr/SetNtcStsCore/NtcNr is Valid/Diagnostics Not Inhibited/NtcEnabled/NTCSTS_FAILD/Update ISO Bits, Parameter Byte and AgiCntr /ProcessRampResponse and DiagcSts/TimedShutdown Fault/Atomic Section2/Update Ramp Rate1 ==
  RampRate : Inport
  Action Port : ActionPort
  CopyRight2 : Subsystem  Description=|  mask(Copyright Information){none=on}
      | Copyright info block.                                               
      |                                                                     
      | Place copyright information at the top of every subsystem in design.
      mask prompts: none "No parameters"
      mask help: Place copyright information at the top of every subsystem in design.
      mask Display:
      | NxtrConf = 'Nexteer Confidential';
      | 
      | sys = bdroot; %handle for the current model ("system")
      | first = get_param(sys,'Created');
      | first = first(end-3:end);  %year is last four digits
      | 
      | last = get_param(sys,'LastModifiedDate');
      | if isempty(last)
      |     last = datestr(now,'yyyy');
      | else
      |     last = last(end-3:end);
      | end
      | 
      | if strcmp(first,last)
      |     fprintf('%s -- Copyright %s Nexteer',NxtrConf,first)
      | else
      |     fprintf('%s -- %s%s- %s Nexteer',NxtrConf,char(169),first,last)
      | end
  ProxySetNtcActvRampRate : Outport
  wires:
  RampRate/1 -> ProxySetNtcActvRampRate/1

== system ES101A_DiagcMgr/DiagcMgr/SetNtcStsCore/NtcNr is Valid/Diagnostics Not Inhibited/NtcEnabled/NTCSTS_FAILD/Update ISO Bits, Parameter Byte and AgiCntr /ProcessRampResponse and DiagcSts/TimedShutdown Fault/Atomic Section2/Update Scale2 ==
  Action Port : ActionPort
  CopyRight2 : Subsystem  Description=|  mask(Copyright Information){none=on}
      | Copyright info block.                                               
      |                                                                     
      | Place copyright information at the top of every subsystem in design.
      mask prompts: none "No parameters"
      mask help: Place copyright information at the top of every subsystem in design.
      mask Display:
      | NxtrConf = 'Nexteer Confidential';
      | 
      | sys = bdroot; %handle for the current model ("system")
      | first = get_param(sys,'Created');
      | first = first(end-3:end);  %year is last four digits
      | 
      | last = get_param(sys,'LastModifiedDate');
      | if isempty(last)
      |     last = datestr(now,'yyyy');
      | else
      |     last = last(end-3:end);
      | end
      | 
      | if strcmp(first,last)
      |     fprintf('%s -- Copyright %s Nexteer',NxtrConf,first)
      | else
      |     fprintf('%s -- %s%s- %s Nexteer',NxtrConf,char(169),first,last)
      | end
  Scale Motor Torque Command to Zero : Constant  Value=SCAMOTTQCMDTOZERO_ULS_F32  OutDataTypeStr=single
  DiagcMgrActvMotTqCmdSca : Outport
  wires:
  Scale Motor Torque Command to Zero/1 -> DiagcMgrActvMotTqCmdSca/1

== system ES101A_DiagcMgr/DiagcMgr/SetNtcStsCore/NtcNr is Valid/Diagnostics Not Inhibited/NtcEnabled/NTCSTS_FAILD/Update ISO Bits, Parameter Byte and AgiCntr /ProcessRampResponse and DiagcSts/TimedShutdown Fault/Atomic Section2/Update Scale3 ==
  Action Port : ActionPort
  CopyRight2 : Subsystem  Description=|  mask(Copyright Information){none=on}
      | Copyright info block.                                               
      |                                                                     
      | Place copyright information at the top of every subsystem in design.
      mask prompts: none "No parameters"
      mask help: Place copyright information at the top of every subsystem in design.
      mask Display:
      | NxtrConf = 'Nexteer Confidential';
      | 
      | sys = bdroot; %handle for the current model ("system")
      | first = get_param(sys,'Created');
      | first = first(end-3:end);  %year is last four digits
      | 
      | last = get_param(sys,'LastModifiedDate');
      | if isempty(last)
      |     last = datestr(now,'yyyy');
      | else
      |     last = last(end-3:end);
      | end
      | 
      | if strcmp(first,last)
      |     fprintf('%s -- Copyright %s Nexteer',NxtrConf,first)
      | else
      |     fprintf('%s -- %s%s- %s Nexteer',NxtrConf,char(169),first,last)
      | end
  Scale Motor Torque Command to Zero : Constant  Value=SCAMOTTQCMDTOZERO_ULS_F32  OutDataTypeStr=single
  ProxySetNtcMotTqCmdSca : Outport
  wires:
  Scale Motor Torque Command to Zero/1 -> ProxySetNtcMotTqCmdSca/1

== system ES101A_DiagcMgr/DiagcMgr/SetNtcStsCore/NtcNr is Valid/Diagnostics Not Inhibited/NtcEnabled/NTCSTS_PREFAILD/Update NtcInfoSts, DebCntr and Process RampRate/DebCntr = MAXDEBCNTRVAL_CNT_S16/Check to Update Snapshot Data/UpdSnpshtData/CopyRight1 ==

== system ES101A_DiagcMgr/DiagcMgr/SetNtcStsCore/NtcNr is Valid/Diagnostics Not Inhibited/NtcEnabled/NTCSTS_PREFAILD/Update NtcInfoSts, DebCntr and Process RampRate/DebCntr = MAXDEBCNTRVAL_CNT_S16/Check to Update Snapshot Data/UpdSnpshtData/Snapshot Data Enabled ==
  NtcNr : Inport
  NtcStInfo : Inport  Port=2
  SnapshotDataBus : Inport  Port=3
  Action Port : ActionPort
  CopyRight2 : Subsystem  Description=|  mask(Copyright Information){none=on}
      | Copyright info block.                                               
      |                                                                     
      | Place copyright information at the top of every subsystem in design.
      mask prompts: none "No parameters"
      mask help: Place copyright information at the top of every subsystem in design.
      mask Display:
      | NxtrConf = 'Nexteer Confidential';
      | 
      | sys = bdroot; %handle for the current model ("system")
      | first = get_param(sys,'Created');
      | first = first(end-3:end);  %year is last four digits
      | 
      | last = get_param(sys,'LastModifiedDate');
      | if isempty(last)
      |     last = datestr(now,'yyyy');
      | else
      |     last = last(end-3:end);
      | end
      | 
      | if strcmp(first,last)
      |     fprintf('%s -- Copyright %s Nexteer',NxtrConf,first)
      | else
      |     fprintf('%s -- %s%s- %s Nexteer',NxtrConf,char(169),first,last)
      | end
  Initialize : Subsystem  Priority=1
      settings: AttributesFormatString=Priority = %<Priority>
  Temp: Snapshot Data Array Index : DataStoreMemory  RequirementInfo={} %GIDa_2572767d_05af_4977_8888_f37035cc543f  DataStoreName=SnpshtDataAryIdx  OutDataTypeStr=uint8  Dimensions=20
  Temp: Snapshot Data Array Index Invalid : DataStoreMemory  RequirementInfo={} %GIDa_64e1585c_9f57_45cc_9f2a_ee713d7d942f  DataStoreName=SnpshtDataAryIdxInvld  InitialValue=1  OutDataTypeStr=boolean  Dimensions=20
  "While " : Subsystem  Priority=2
      settings: AttributesFormatString=Priority = %<Priority>
  wires:
  NtcNr/1 -> "While "/1(NtcNr)
  NtcStInfo/1 -> "While "/2(NtcStInfo)
  SnapshotDataBus/1 -> "While "/3(SnapshotDataBus)
